simulink model "multiple_models"  (R2016a)
settings: Solver=VariableStepAuto  StartTime=0.0  StopTime=10.0  RelTol=1e-3
settings Model: Creator=Pichau  LastModifiedBy=Pichau

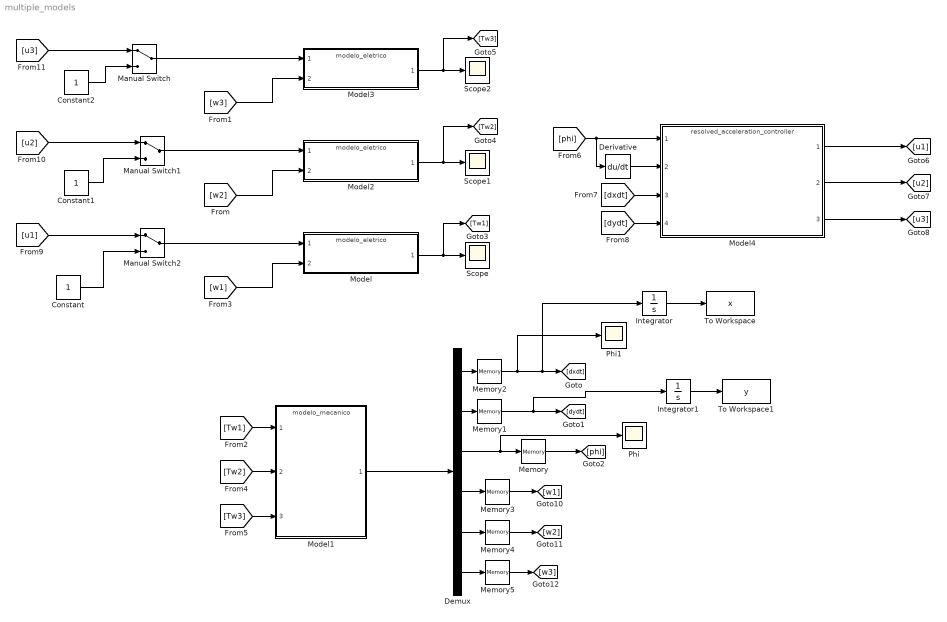
== system multiple_models ==
  Constant : Constant
  Constant1 : Constant
  Constant2 : Constant
  Demux : Demux  Outputs=6
  Derivative : Derivative
  Integrator : Integrator  InitialCondition=0.3
  Integrator1 : Integrator
  Manual Switch : ManualSwitch
  Manual Switch1 : ManualSwitch
  Manual Switch2 : ManualSwitch
  Memory : Memory  X0=pi/2
  Memory{1..5} (5 alike) : Memory
  Model : ModelReference  ModelNameDialog=modelo_eletrico.slx  SimulationMode=Normal  ModelReferenceVersion=1.22
  Model1 : ModelReference  ModelNameDialog=modelo_mecanico.slx  SimulationMode=Normal  ModelReferenceVersion=1.2
  Model2 : ModelReference  ModelNameDialog=modelo_eletrico.slx  SimulationMode=Normal  ModelReferenceVersion=1.22
  Model3 : ModelReference  ModelNameDialog=modelo_eletrico.slx  SimulationMode=Normal  ModelReferenceVersion=1.22
  Model4 : ModelReference  ModelNameDialog=resolved_acceleration_controller.slx  SimulationMode=Normal  ModelReferenceVersion=1.9
  Phi : Scope
  Phi1 : Scope
  Scope : Scope
  Scope1 : Scope
  Scope2 : Scope
  To Workspace : ToWorkspace  VariableName=x  SaveFormat=Timeseries  SampleTime=-1
  To Workspace1 : ToWorkspace  VariableName=y  SaveFormat=Timeseries  SampleTime=-1
  wires:
  Manual Switch2/1 -> Model/1
  Model/1 -> [Tw1], Scope/1
  Demux/3 -> Memory/1, Phi/1
  Demux/4 -> Memory3/1
  Demux/5 -> Memory4/1
  Demux/6 -> Memory5/1
  Demux/1 -> Memory2/1
  Demux/2 -> Memory1/1
  [w1] -> Model/2
  Manual Switch1/1 -> Model2/1
  [w2] -> Model2/2
  [u3] -> Manual Switch/1
  [w3] -> Model3/2
  Model2/1 -> [Tw2], Scope1/1
  Model3/1 -> [Tw3], Scope2/1
  [Tw1] -> Model1/1
  [Tw3] -> Model1/3
  [Tw2] -> Model1/2
  Derivative/1 -> Model4/2
  [phi] -> Model4/1, Derivative/1
  [dxdt] -> Model4/3
  [dydt] -> Model4/4
  Model4/1 -> [u1]
  Model4/2 -> [u2]
  Model4/3 -> [u3]
  Model1/1 -> Demux/1
  Memory/1 -> [phi]
  Memory1/1 -> Integrator1/1, [dydt]
  Memory2/1 -> Phi1/1, Integrator/1, [dxdt]
  Memory3/1 -> [w1]
  Memory4/1 -> [w2]
  Memory5/1 -> [w3]
  Manual Switch/1 -> Model3/1
  [u2] -> Manual Switch1/1
  [u1] -> Manual Switch2/1
  Constant/1 -> Manual Switch2/2
  Constant1/1 -> Manual Switch1/2
  Constant2/1 -> Manual Switch/2
  Integrator/1 -> To Workspace/1
  Integrator1/1 -> To Workspace1/1
